simulink model "BasicModel"  (Simulink 7.7)
settings: Solver=ode45  StartTime=0.0  StopTime=Inf  RelTol=1e-3
libraries: vrlib x1
settings Model: Creator=Artem  LastModifiedBy=Artem

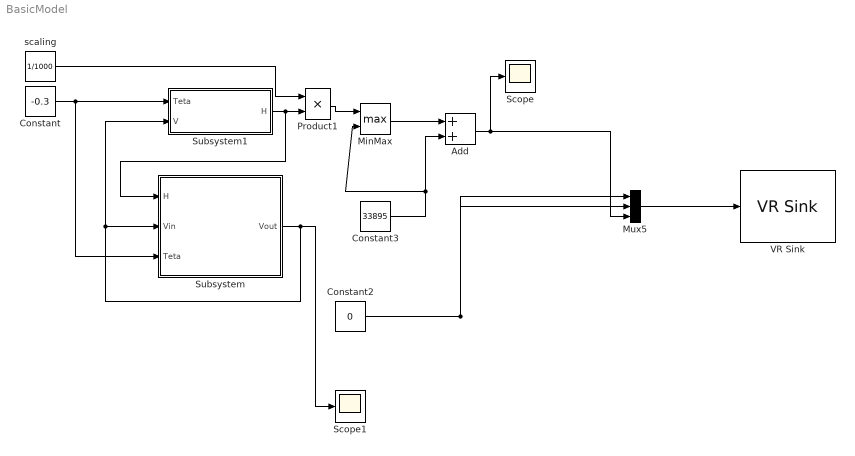
== system BasicModel ==
  Add : Sum
  Constant : Constant  Value=-0.3
  Constant2 : Constant  Value=0
  Constant3 : Constant  Value=33895
  MinMax : MinMax  Function=max  Inputs=2
  Mux5 : Mux  Inputs=3
  Product1 : Product  RndMeth=Zero
  Scope : Scope
      settings: YMin=73.89  YMax=73.99
  Scope1 : Scope
  Subsystem : Subsystem
  Subsystem1 : Subsystem
  VR Sink : vrlib/VR Sink  SampleTime=0.1  ViewEnable=on  RemoteChange=off  RemoteView=on  FieldsWritten=Ship.translation.3.1.1.double  WorldFileName=vrplanets.wrl  WorldDescription=Planets  AutoView=off  VideoDimensions=[]  FigureProperties="{'Position', 'Name', 'Viewpoint', 'CameraBound', 'CameraDirection', 'CameraPosition', 'CameraUpVector', 'ZoomFactor', 'Antialiasing', 'Headlight', 'Lighting', 'NavPanel', 'StatusBar', 'ToolBar', 'Textures', 'Transparency', 'Wireframe', 'NavZones', 'NavMode', 'NavSpeed', 'Record2DCompressMethod', 'Record2DCompressQuality', 'Record2D', 'Record2DFileName', 'Record2DFPS'; [4.3600000000000000e+002  5.7800000000000000e+002  5.7600000000000000e+002  3.8000000000000000e+002], 'Planets', '_untitled_4', 'on', [2.7769161882744847e-001  9.3459051871211521e-002 -9.5611336694783355e-001], [0.0000000000000000e+000  0.0000000000000000e+000  0.0000000000000000e+000], [7.7767428529828972e-002  9.8980325026807014e-001  1.1933881522212664e-001], [1.0000000000000000e+000], 'on', 'off', 'on', 'halfbar', 'on', 'on', 'on', 'on', 'off', 'off', 'fly', 'normal', 'auto', [7.5000000000000000e+001], 'off', '%f_anim_%n.avi', [1.5000000000000000e+001]}"
  scaling : Constant  Value=1/1000
  wires:
  Constant/1 -> Subsystem1/1(Teta), Subsystem/3(Teta)
  Subsystem1/1(H) -> Subsystem/1(H), Product1/2
  Subsystem/1(Vout) -> Subsystem/2(Vin), Subsystem1/2(V), Scope1/1
  Mux5/1 -> VR Sink/1
  Constant2/1 -> Mux5/1, Mux5/2
  Constant3/1 -> Add/2, MinMax/2
  MinMax/1 -> Add/1
  Product1/1 -> MinMax/1
  Add/1 -> Mux5/3, Scope/1
  scaling/1 -> Product1/1

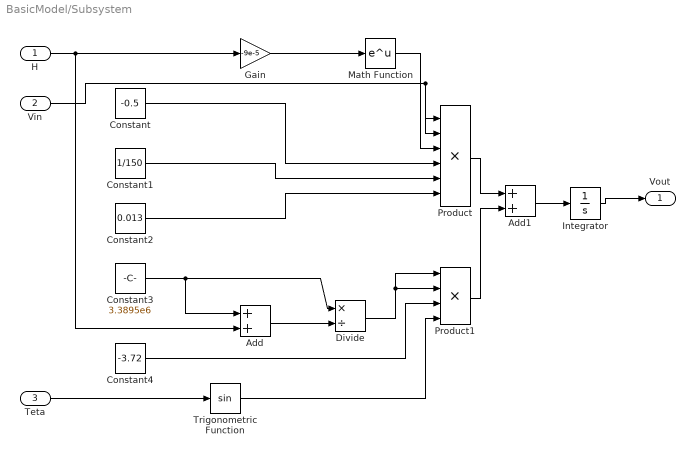
== system BasicModel/Subsystem ==
  H : Inport
  Vin : Inport  Port=2
  Teta : Inport  Port=3
  Add : Sum
  Add1 : Sum
  Constant : Constant  Value=-0.5
  Constant1 : Constant  Value=1/150
  Constant2 : Constant  Value=0.013
  Constant3 : Constant  Value=3.3895e6
  Constant4 : Constant  Value=-3.72
  Divide : Product  Inputs=*/
  Gain : Gain  Gain=-9e-5
  Integrator : Integrator  InitialCondition=20  ContinuousStateAttributes='height'
  Math Function : Math  SaturateOnIntegerOverflow=on
  Product : Product  Inputs=6  RndMeth=Zero
  Product1 : Product  Inputs=4  RndMeth=Zero
  Trigonometric Function : Trigonometry
  Vout : Outport
  wires:
  H/1 -> Add/2, Gain/1
  Constant3/1 -> Add/1, Divide/1
  Add/1 -> Divide/2
  Constant/1 -> Product/4
  Constant1/1 -> Product/5
  Constant2/1 -> Product/6
  Vin/1 -> Product/1, Product/2
  Gain/1 -> Math Function/1
  Math Function/1 -> Product/3
  Product/1 -> Add1/1
  Product1/1 -> Add1/2
  Add1/1 -> Integrator/1
  Integrator/1 -> Vout/1
  Divide/1 -> Product1/2, Product1/1
  Constant4/1 -> Product1/3
  Teta/1 -> Trigonometric Function/1
  Trigonometric Function/1 -> Product1/4

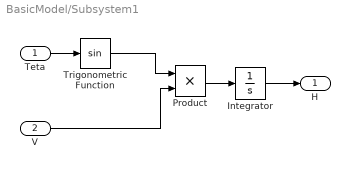
== system BasicModel/Subsystem1 ==
  Teta : Inport
  V : Inport  Port=2
  Integrator : Integrator  InitialCondition=244000  LowerSaturationLimit=0  ContinuousStateAttributes='velocity'
  Product : Product  RndMeth=Zero
  Trigonometric Function : Trigonometry
  H : Outport
  wires:
  V/1 -> Product/2
  Teta/1 -> Trigonometric Function/1
  Trigonometric Function/1 -> Product/1
  Product/1 -> Integrator/1
  Integrator/1 -> H/1
